simulink model "Practica_1_Representacion_A_Bloques_De_Ecuaciones_Diferenciales_En_Simulink_HERNANDEZ_GONZALEZ_ALEJANDRO"  (R2026a)
settings: Solver=VariableStepAuto
PreLoadFcn:
  | Ip = 0.0079;
  | Mc = 0.7031;
  | lp = 0.3302;
  | Mp = 0.23;
  | Fc = 0;
  | Beq = 4.3;
  | g = 9.81;
  | Bp = 0.0024;
settings Model: Creator=Alejandro  LastModifiedBy=Alejandro

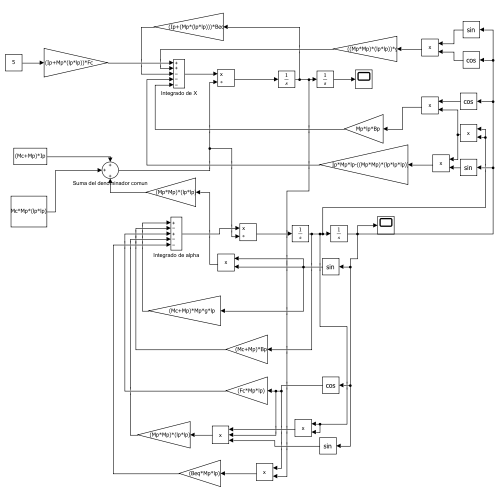
[thumbnail: Simulink's stored preview of the top-level diagram]
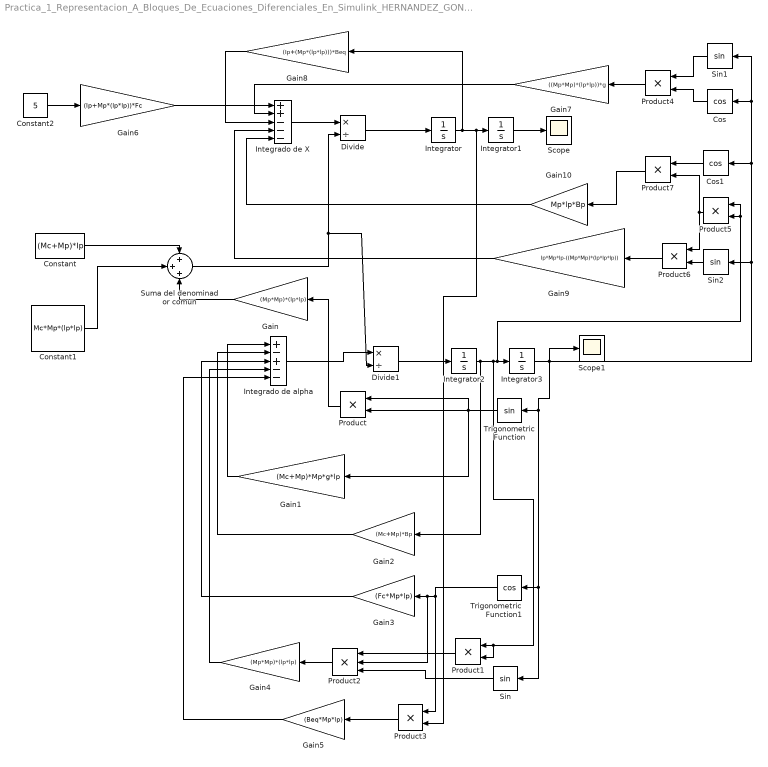
== system Practica_1_Representacion_A_Bloques_De_Ecuaciones_Diferenciales_En_Simulink_HERNANDEZ_GONZALEZ_ALEJANDRO ==
  Constant : Constant  Value=(Mc+Mp)*Ip
  Constant1 : Constant  Value=Mc*Mp*(lp*lp)
  Constant2 : Constant  Value=5
  Cos : Trigonometry  Operator=cos
  Cos1 : Trigonometry  Operator=cos
  Divide : Product  Inputs=*/
  Divide1 : Product  Inputs=*/
  Gain : Gain  Gain=(Mp*Mp)*(lp*lp)
  Gain1 : Gain  Gain=(Mc+Mp)*Mp*g*lp
  Gain10 : Gain  Gain=Mp*lp*Bp
  Gain2 : Gain  Gain=(Mc+Mp)*Bp
  Gain3 : Gain  Gain=(Fc*Mp*lp)
  Gain4 : Gain  Gain=(Mp*Mp)*(lp*lp)
  Gain5 : Gain  Gain=(Beq*Mp*lp)
  Gain6 : Gain  Gain=(Ip+Mp*(lp*lp))*Fc
  Gain7 : Gain  Gain=((Mp*Mp)*(lp*lp))*g
  Gain8 : Gain  Gain=(Ip+(Mp*(lp*lp)))*Beq
  Gain9 : Gain  Gain=Ip*Mp*lp-((Mp*Mp)*(lp*lp*lp))
  Integrado de X : Sum  Inputs=++---
  Integrado de alpha : Sum  Inputs=+-+--
  Integrator : Integrator
  Integrator1 : Integrator  InitialCondition=0.1
  Integrator2 : Integrator
  Integrator3 : Integrator  InitialCondition=1*pi/180
  Product{,1,3..7} (7 alike) : Product
  Product2 : Product  Inputs=3
  Scope : Scope
      settings: ActiveDisplayYMinimum=-0.56745392976464526  ActiveDisplayYMaximum=0.97702536312985266
  Scope1 : Scope
      settings: ActiveDisplayYMinimum=-65.27246848378168  ActiveDisplayYMaximum=147.59915043100949
  Sin : Trigonometry
  Sin1 : Trigonometry
  Sin2 : Trigonometry
  Suma del denominador comun : Sum  Inputs=+++
  Trigonometric Function : Trigonometry
  Trigonometric Function1 : Trigonometry  Operator=cos
  wires:
  Integrator/1 -> Gain8/1, Integrator1/1, Product3/2
  Integrator3/1 -> Cos1/1, Sin1/1, Cos/1, Sin2/1, Trigonometric Function1/1, Sin/1, Trigonometric Function/1, Scope1/1
  Integrator2/1 -> Gain2/1, Product5/1, Product5/2, Integrator3/1, Product1/2, Product1/1
  Integrator1/1 -> Scope/1
  Divide/1 -> Integrator/1
  Constant/1 -> Suma del denominador comun/1
  Constant1/1 -> Suma del denominador comun/2
  Trigonometric Function/1 -> Gain1/1, Product/1, Product/2
  Product/1 -> Gain/1
  Gain/1 -> Suma del denominador comun/3
  Suma del denominador comun/1 -> Divide1/2, Divide/2
  Integrado de X/1 -> Divide/1
  Divide1/1 -> Integrator2/1
  Integrado de alpha/1 -> Divide1/1
  Gain1/1 -> Integrado de alpha/1
  Gain2/1 -> Integrado de alpha/2
  Trigonometric Function1/1 -> Product3/1, Product2/2, Gain3/1
  Gain3/1 -> Integrado de alpha/3
  Product1/1 -> Product2/1
  Product2/1 -> Gain4/1
  Gain4/1 -> Integrado de alpha/4
  Sin/1 -> Product2/3
  Product3/1 -> Gain5/1
  Gain5/1 -> Integrado de alpha/5
  Gain6/1 -> Integrado de X/1
  Constant2/1 -> Gain6/1
  Sin1/1 -> Product4/1
  Product4/1 -> Gain7/1
  Cos/1 -> Product4/2
  Gain7/1 -> Integrado de X/2
  Gain8/1 -> Integrado de X/3
  Product5/1 -> Product6/1, Product7/2
  Sin2/1 -> Product6/2
  Product6/1 -> Gain9/1
  Gain9/1 -> Integrado de X/4
  Cos1/1 -> Product7/1
  Product7/1 -> Gain10/1
  Gain10/1 -> Integrado de X/5
